simulink model "PMSM_PI_decomposition_Discrete_Time"  (R2024a)
settings: Solver=ode23tb  StartTime=0.0  StopTime=10  FixedStep=0.0002  RelTol=1e-4  EnableMultiTasking=on
InitFcn:
  | Ts = 10e-6;
  | 
  | R = 0.958;
  | Ld = 5.25e-3;
  | Lq = 12e-3;
  | Pn = 4;
  | flux = 0.1827;
values from neighbouring files (symbols this model uses):
  Flux = 0.1827    [Parameters.m]    (also in StateSpace.m = 0.192)
  Ki = (Ld*2*pi*fsw)/10    (= 2.4975661596)    [StateSpace.m]
  Kp = (Lq*2*pi*fsw)/10    (= 2.4975661596)    [StateSpace.m]
  L_d = 0.00525    [Parameters.m]
  L_q = 0.00525    [Parameters.m]
  p = 4    [Parameters.m]    (also in StateSpace.m)
  R_s = 0.9585    [Parameters.m]
undefined symbols (not defined in the file or in its folder): DiscIntNeverNeededParam, Ki_s, Kp_s
libraries: simulink x2, spsPermanentMagnetSynchronousMachineLib x1, spsUniversalBridgeLib x1, spsDCVoltageSourceLib x1, sps_lib x1
settings Model: Creator=SUN  LastModifiedBy=nicco
settings SolverCC: ZeroCrossControl=DisableAll  AlgebraicLoopSolver=TrustRegion
settings DataIOCC: LimitDataPoints=on  SaveFormat=Array  SignalLoggingSaveFormat=ModelDataLogs  ReturnWorkspaceOutputs=off
settings OptimizationCC: ExpressionDepthLimit=2147483647  InitFltsAndDblsToZero=on  LifeSpan=inf
settings DebuggingCC: UnderspecifiedInitializationDetection=Classic  MergeDetectMultiDrivingBlocksExec=none  SolverPrmCheckMsg=warning  FcnCallInpInsideContextMsg=warning  UnconnectedInputMsg=warning  UnconnectedOutputMsg=warning  UnconnectedLineMsg=warning  StateNameClashWarn=warning  SFUnexpectedBacktrackingDiag=warning  SFNoUnconditionalDefaultTransitionDiag=warning  SFExecutionAtInitializationDiag=none  ArithmeticOperatorsInVariantConditions=warning
settings HardwareCC: ProdBitPerPointer=32  ProdBitPerSizeT=32  ProdBitPerPtrDiffT=32  ProdLargestAtomicFloat=None  ProdIntDivRoundTo=Undefined  ProdEndianess=Unspecified  ProdWordSize=32  ProdHWDeviceType=32-bit Generic
settings ModelReferenceCC: EnableRefExpFcnMdlSchedulingChecks=on  PropagateSignalLabelsOutOfModel=off
settings SFSimCC: SimUseLocalCustomCode=off  CustomCodeUndefinedFunction=UseInterfaceOnly
settings RTWCC: RTWUseLocalCustomCode=off  GPUComputeCapability=3.5
settings CodeAppCC: StateflowObjectComments=on
settings GRTTargetCC: TargetLangStandard=C89/C90 (ANSI)  CombineOutputUpdateFcns=off  GRTInterface=on
settings ConfigComp: CovMetricSettings=dw  CovSaveCumulativeToWorkspaceVar=on  CovSaveSingleToWorkspaceVar=on  CovExternalEMLEnable=off  CovSFcnEnable=off
settings SimscapeCC: SimscapeNormalizeSystem=off

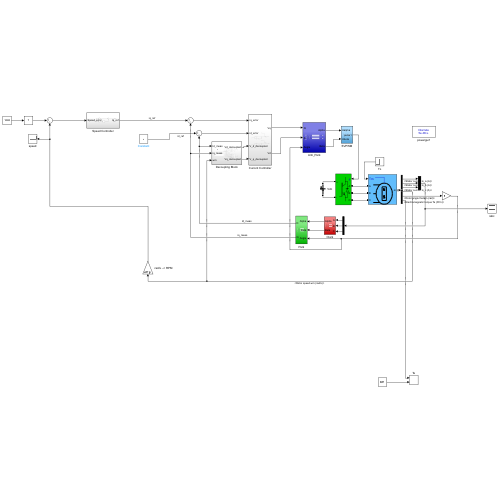
[thumbnail: Simulink's stored preview of the top-level diagram]
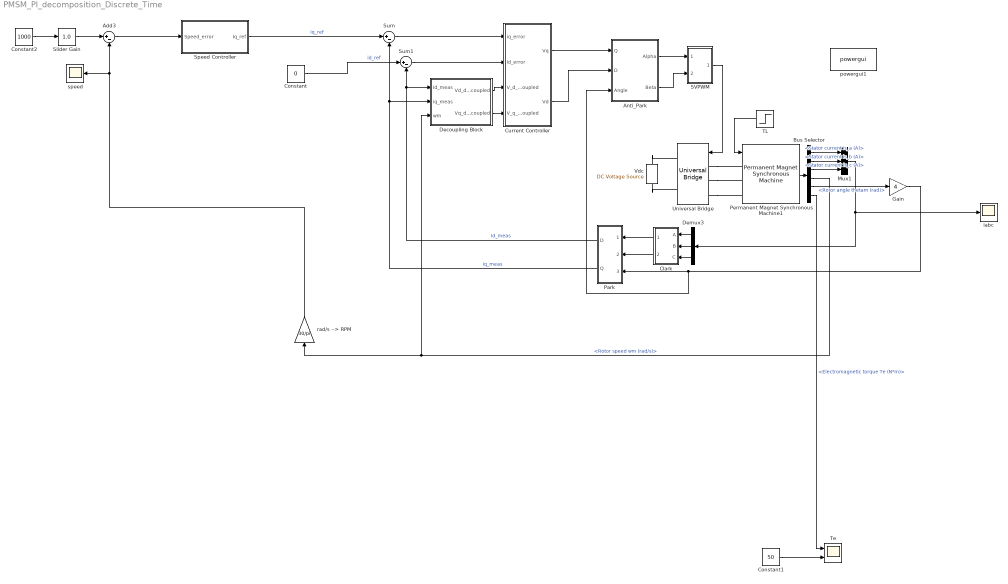
== system PMSM_PI_decomposition_Discrete_Time ==
  Add3 : Sum  Inputs=|+-
  Anti_Park : Subsystem
  Bus Selector : BusSelector  OutputSignals=Stator current is_a (A),Stator current is_b (A),Stator current is_c (A),Rotor speed wm (rad/s),Rotor angle thetam (rad),Electromagnetic torque Te (N*m)
  Clark : Subsystem
  Constant : Constant  Value=0
  Constant1 : Constant  Value=50
  Constant2 : Constant  Value=1000
  Current Controller : Subsystem
  Decoupling Block : Subsystem
  Demux3 : Demux  Outputs=3
  Gain : Gain  Gain=4
  Mux1 : Mux  Inputs=3
  Park : Subsystem
  Permanent Magnet Synchronous Machine1 : spsPermanentMagnetSynchronousMachineLib/Permanent Magnet Synchronous Machine  NbPhases=3  FluxDistribution=Sinusoidal  RotorType=Salient-pole  MechanicalLoad=Torque Tm  PresetModel=No  ShowDetailedParameters=on  MeasurementBus=off  Resistance=R_s  Inductance=8.5e-3  dqInductances=[L_d L_q]  La=L_d  MachineConstant=Flux linkage established by magnets (V.s)  Flux=Flux  VoltageCst=132.5525  TorqueCst=1.0962  Flat=120  Mechanical=[0.003 0.008 p]  PolePairs=3  InitialConditions=[0,0, 0,0]  InitialConditions5ph=[0 0 0 0 0 0]  RefAngle=Aligned with phase A axis (original Park)  IterativeDiscreteModel=Trapezoidal non iterative  TsBlock=-1  TsPowergui=0
  SVPWM : Subsystem
  Slider Gain : simulink/Math Operations/Slider Gain  gain=1.0  low=0  high=2
  Speed Controller : Subsystem
  Sum : Sum  Inputs=|+-
  Sum1 : Sum  Inputs=|+-
  TL : Step  Time=0.2  After=0  SampleTime=0
  Te : Scope  NumInputPorts=2
  Universal Bridge : spsUniversalBridgeLib/Universal Bridge  Arms=3  SnubberResistance=1e5  SnubberCapacitance=inf  Device=IGBT / Diodes  Ron=1e-3  Lon=0  ForwardVoltages="[  0  0  ]"  ForwardVoltage=0  GTOparameters=[ 10e-6 , 20e-6 ]  IGBTparameters=[ 1e-6 , 2e-6 ]  Measurements=None  Measurements_2=None  converterType=Rectifier
  Vdc : spsDCVoltageSourceLib/DC Voltage Source  Amplitude=600  Measurements=None
  iabc : Scope
  powergui1 : sps_lib/powergui  Priority=1  SimulationMode=Discrete  SampleTime=5e-6  frequency=60  Iterations=50  frequencyindice=0  Pbase=100e6  ErrMax=1e-4  UnitsV=kV  UnitsW=MW  buscounter=0  FunctionMessages=off  echomessages=off  EnableUseOfTLC=off  CurrentSourceSwitches=off  DisableSnubberDevices=off  DisableRonSwitches=off  DisableVfSwitches=off  DisplayEquations=off  AutomaticDiscreteSolvers=off  SolverType=Tustin/Backward Euler (TBE)  Interpol=off  ExternalGateDelay=off  methode=off  Ts=100  x0status=blocks  SPID=on  SwTol=0  HookPort=off  NonlinearTolerance=1e-4  nMaxIteration=100  ContinueOnMaxIteration=off  RestoreLinks=warning  ResistiveCurrentMeasurement=off  Frange=[0:2:500]  Ylog=off  Xlog=on  ShowGrid=off  save=off  variable=ZData  structure=0  ZoomFFT=off  StartTime=0.0  cycles=1  DisplayStyle=1  fundamental=60  FreqAxis=off  MaxFrequency=1000  frequencyindicesteady=1  RmsSteady=1  display=off
  rad/s --> RPM : Gain  Gain=30/pi
  speed : Scope
  wires:
  TL/1 -> Permanent Magnet Synchronous Machine1/1
  Gain/1 -> Park/3(Angle), Anti_Park/3(Angle)
  Anti_Park/1(Alpha) -> SVPWM/1(Ualpha)
  Demux3/1 -> Clark/1(A)
  Anti_Park/2(Beta) -> SVPWM/2(Ubeta)
  Demux3/2 -> Clark/2(B)
  Demux3/3 -> Clark/3(C)
  Clark/1(Alpha) -> Park/1(Alpha)
  Clark/2(Beta) -> Park/2(Beta)
  Bus Selector/3 -> Mux1/3  "<Stator current is_c (A)>"
  Bus Selector/2 -> Mux1/2  "<Stator current is_b (A)>"
  Bus Selector/1 -> Mux1/1  "<Stator current is_a (A)>"
  Mux1/1 -> iabc/1, Demux3/1
  Permanent Magnet Synchronous Machine1/1 -> Bus Selector/1
  Bus Selector/5 -> Gain/1  "<Rotor angle thetam (rad)>"
  Bus Selector/6 -> Te/1  "<Electromagnetic torque Te (N*m)>"
  SVPWM/1(pulse1) -> Universal Bridge/1
  Constant/1 -> Sum1/1  "id_ref"
  Sum/1 -> Current Controller/1(iq_error)
  Park/2(Q) -> Sum/2, Decoupling Block/2(iq_meas)  "iq_meas"
  Decoupling Block/2(Vq_decoupled) -> Current Controller/4(V_q_decoupled)
  Park/1(D) -> Sum1/2, Decoupling Block/1(Id_meas)  "Id_meas"
  Sum1/1 -> Current Controller/2(id_error)
  Decoupling Block/1(Vd_decoupled) -> Current Controller/3(V_d_decoupled)
  Bus Selector/4 -> Decoupling Block/3(wm), rad/s --> RPM/1  "<Rotor speed wm (rad/s)>"
  Current Controller/2(Vd) -> Anti_Park/2(D)
  Current Controller/1(Vq) -> Anti_Park/1(Q)
  Slider Gain/1 -> Add3/1
  rad/s --> RPM/1 -> Add3/2, speed/1
  Constant1/1 -> Te/2
  Speed Controller/1(Iq_ref) -> Sum/1  "iq_ref"
  Add3/1 -> Speed Controller/1(Speed_error)
  Constant2/1 -> Slider Gain/1
  connections:
  Universal Bridge/LConn1 -- Permanent Magnet Synchronous Machine1/LConn1
  Universal Bridge/LConn2 -- Permanent Magnet Synchronous Machine1/LConn2
  Universal Bridge/LConn3 -- Permanent Magnet Synchronous Machine1/LConn3
  Vdc/RConn1 -- Universal Bridge/RConn1
  Vdc/LConn1 -- Universal Bridge/RConn2

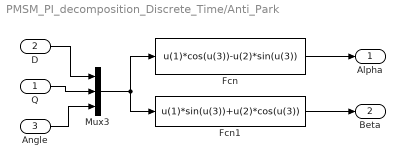
== system PMSM_PI_decomposition_Discrete_Time/Anti_Park ==
  Q : Inport
  D : Inport  Port=2
  Angle : Inport  Port=3
  Fcn : Fcn  Expr=u(1)*cos(u(3))-u(2)*sin(u(3))
  Fcn1 : Fcn  Expr=u(1)*sin(u(3))+u(2)*cos(u(3))
  Mux3 : Mux  Inputs=3
  Alpha : Outport  VectorParamsAs1DForOutWhenUnconnected=off
  Beta : Outport  Port=2  VectorParamsAs1DForOutWhenUnconnected=off
  wires:
  Angle/1 -> Mux3/3
  Fcn1/1 -> Beta/1
  Mux3/1 -> Fcn1/1, Fcn/1
  Fcn/1 -> Alpha/1
  D/1 -> Mux3/1
  Q/1 -> Mux3/2

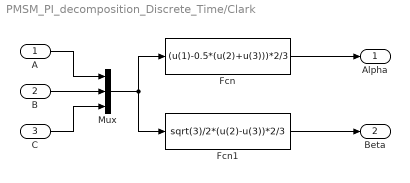
== system PMSM_PI_decomposition_Discrete_Time/Clark ==
  A : Inport
  B : Inport  Port=2
  C : Inport  Port=3
  Fcn : Fcn  Expr=(u(1)-0.5*(u(2)+u(3)))*2/3
  Fcn1 : Fcn  Expr=sqrt(3)/2*(u(2)-u(3))*2/3
  Mux : Mux  Inputs=3
  Alpha : Outport  VectorParamsAs1DForOutWhenUnconnected=off
  Beta : Outport  Port=2  VectorParamsAs1DForOutWhenUnconnected=off
  wires:
  B/1 -> Mux/2
  Mux/1 -> Fcn1/1, Fcn/1
  Fcn1/1 -> Beta/1
  Fcn/1 -> Alpha/1
  C/1 -> Mux/3
  A/1 -> Mux/1

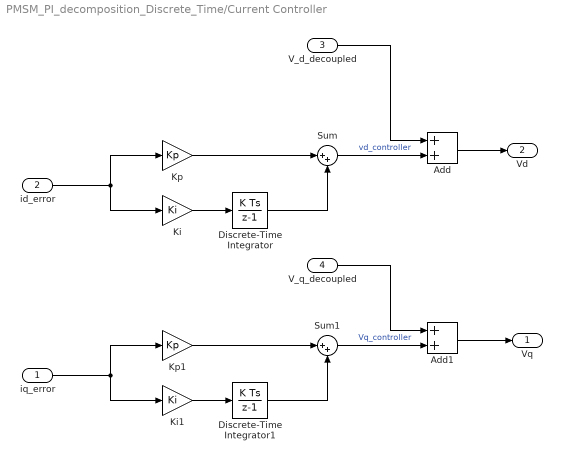
== system PMSM_PI_decomposition_Discrete_Time/Current Controller ==
  iq_error : Inport
  id_error : Inport  Port=2
  V_d_decoupled : Inport  Port=3
  V_q_decoupled : Inport  Port=4
  Add : Sum
  Add1 : Sum
  Discrete-Time Integrator : DiscreteIntegrator  SampleTime=-1  ICPrevOutput=DiscIntNeverNeededParam  ICPrevScaledInput=DiscIntNeverNeededParam
  Discrete-Time Integrator1 : DiscreteIntegrator  SampleTime=-1  ICPrevOutput=DiscIntNeverNeededParam  ICPrevScaledInput=DiscIntNeverNeededParam
  Ki : Gain  Gain=Ki
  Ki1 : Gain  Gain=Ki
  Kp : Gain  Gain=Kp
  Kp1 : Gain  Gain=Kp
  Sum : Sum  Inputs=|++
  Sum1 : Sum  Inputs=|++
  Vq : Outport
  Vd : Outport  Port=2
  wires:
  Add/1 -> Vd/1
  id_error/1 -> Ki/1, Kp/1
  V_q_decoupled/1 -> Add1/1
  Ki1/1 -> Discrete-Time Integrator1/1
  V_d_decoupled/1 -> Add/1
  iq_error/1 -> Ki1/1, Kp1/1
  Kp1/1 -> Sum1/1
  Sum/1 -> Add/2  "vd_controller"
  Sum1/1 -> Add1/2  "Vq_controller"
  Discrete-Time Integrator1/1 -> Sum1/2
  Discrete-Time Integrator/1 -> Sum/2
  Ki/1 -> Discrete-Time Integrator/1
  Kp/1 -> Sum/1
  Add1/1 -> Vq/1

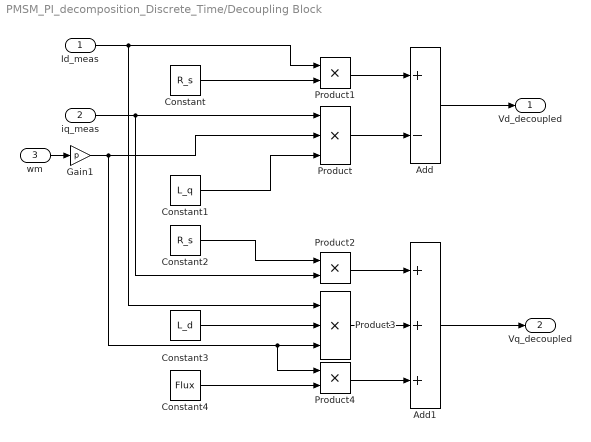
== system PMSM_PI_decomposition_Discrete_Time/Decoupling Block ==
  Id_meas : Inport
  iq_meas : Inport  Port=2
  wm : Inport  Port=3
  Add : Sum  Inputs=+-
  Add1 : Sum  Inputs=+++
  Constant : Constant  Value=R_s
  Constant1 : Constant  Value=L_q
  Constant2 : Constant  Value=R_s
  Constant3 : Constant  Value=L_d
  Constant4 : Constant  Value=Flux
  Gain1 : Gain  Gain=p
  Product : Product  Inputs=3
  Product1 : Product
  Product2 : Product
  Product3 : Product  Inputs=3
  Product4 : Product
  Vd_decoupled : Outport
  Vq_decoupled : Outport  Port=2
  wires:
  Add/1 -> Vd_decoupled/1
  Product1/1 -> Add/1
  Constant/1 -> Product1/2
  Id_meas/1 -> Product1/1, Product3/1
  Product/1 -> Add/2
  Gain1/1 -> Product4/1, Product3/3, Product/2
  Constant1/1 -> Product/3
  Add1/1 -> Vq_decoupled/1
  Product2/1 -> Add1/1
  Constant2/1 -> Product2/1
  iq_meas/1 -> Product/1, Product2/2
  Product3/1 -> Add1/2
  Constant3/1 -> Product3/2
  Product4/1 -> Add1/3
  Constant4/1 -> Product4/2
  wm/1 -> Gain1/1

== system PMSM_PI_decomposition_Discrete_Time/Park ==
  Alpha : Inport
  Beta : Inport  Port=2
  Angle : Inport  Port=3
  Fcn : Fcn  Expr=u(1)*cos(u(3))+u(2)*sin(u(3))
  Fcn1 : Fcn  Expr=u(2)*cos(u(3))-u(1)*sin(u(3))
  Mux2 : Mux  Inputs=3
  D : Outport  VectorParamsAs1DForOutWhenUnconnected=off
  Q : Outport  Port=2  VectorParamsAs1DForOutWhenUnconnected=off
  wires:
  Beta/1 -> Mux2/2
  Mux2/1 -> Fcn1/1, Fcn/1
  Angle/1 -> Mux2/3
  Alpha/1 -> Mux2/1
  Fcn1/1 -> Q/1
  Fcn/1 -> D/1

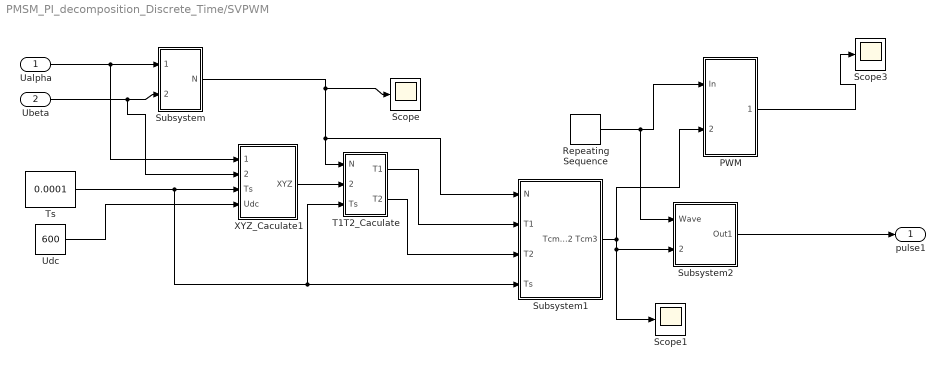
== system PMSM_PI_decomposition_Discrete_Time/SVPWM ==
  Ualpha : Inport
  Ubeta : Inport  Port=2
  PWM : Subsystem
  Repeating Sequence : simulink/Sources/Repeating Sequence  rep_seq_t=[0 0.00005 0.0001]  rep_seq_y=[0 0.00005 0]
  Scope : Scope
  Scope1 : Scope
  Scope3 : Scope
  Subsystem : Subsystem
  Subsystem1 : Subsystem
  Subsystem2 : Subsystem
  T1T2_Caculate : Subsystem
  Ts : Constant  Value=0.0001
  Udc : Constant  Value=600
  XYZ_Caculate1 : Subsystem
  pulse1 : Outport  VectorParamsAs1DForOutWhenUnconnected=off
  wires:
  T1T2_Caculate/1(T1) -> Subsystem1/2(T1)
  Ts/1 -> XYZ_Caculate1/3(Ts), T1T2_Caculate/3(Ts), Subsystem1/4(Ts)
  Udc/1 -> XYZ_Caculate1/4(Udc)
  Subsystem/1(N) -> Scope/1, T1T2_Caculate/1(N), Subsystem1/1(N)
  T1T2_Caculate/2(T2) -> Subsystem1/3(T2)
  XYZ_Caculate1/1("XYZ ") -> T1T2_Caculate/2(XYZ)
  Ualpha/1 -> XYZ_Caculate1/1(Ualpha), Subsystem/1(Ualpha)
  Ubeta/1 -> XYZ_Caculate1/2(Ubeta), Subsystem/2(Ubeta)
  Subsystem1/1(Tcm1 Tcm2 Tcm3) -> Scope1/1, Subsystem2/2(Tcm123), PWM/2(Tcm123)
  Repeating Sequence/1 -> Subsystem2/1(Wave), PWM/1(In)
  PWM/1(PWM) -> Scope3/1
  Subsystem2/1(Out1) -> pulse1/1

== system PMSM_PI_decomposition_Discrete_Time/Speed Controller ==
  Speed_error : Inport
  Discrete-Time Integrator : DiscreteIntegrator  SampleTime=-1  ICPrevOutput=DiscIntNeverNeededParam  ICPrevScaledInput=DiscIntNeverNeededParam
  Ki : Gain  Gain=Ki_s
  Kp : Gain  Gain=Kp_s
  Sum2 : Sum  Inputs=|++
  Iq_ref : Outport
  wires:
  Discrete-Time Integrator/1 -> Sum2/2
  Sum2/1 -> Iq_ref/1  "vd_controller"
  Kp/1 -> Sum2/1
  Speed_error/1 -> Ki/1, Kp/1
  Ki/1 -> Discrete-Time Integrator/1

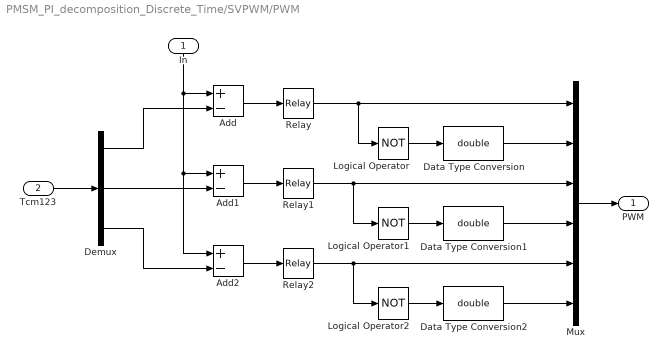
== system PMSM_PI_decomposition_Discrete_Time/SVPWM/PWM ==
  In : Inport
  Tcm123 : Inport  Port=2
  Add : Sum  Inputs=+-
  Add1 : Sum  Inputs=+-
  Add2 : Sum  Inputs=+-
  Data Type Conversion : DataTypeConversion  OutDataTypeStr=double  SaturateOnIntegerOverflow=off  RndMeth=Floor
  Data Type Conversion1 : DataTypeConversion  OutDataTypeStr=double  SaturateOnIntegerOverflow=off  RndMeth=Floor
  Data Type Conversion2 : DataTypeConversion  OutDataTypeStr=double  SaturateOnIntegerOverflow=off  RndMeth=Floor
  Demux : Demux  Outputs=3
  Logical Operator : Logic  Operator=NOT  AllPortsSameDT=off  OutDataTypeStr=boolean
  Logical Operator1 : Logic  Operator=NOT  AllPortsSameDT=off  OutDataTypeStr=boolean
  Logical Operator2 : Logic  Operator=NOT  AllPortsSameDT=off  OutDataTypeStr=boolean
  Mux : Mux  Inputs=6
  Relay : Relay  OffSwitchValue=-eps
  Relay1 : Relay  OffSwitchValue=-eps
  Relay2 : Relay  OffSwitchValue=-eps
  PWM : Outport  VectorParamsAs1DForOutWhenUnconnected=off
  wires:
  Demux/3 -> Add2/2
  Demux/2 -> Add1/2
  Demux/1 -> Add/2
  Relay2/1 -> Mux/5, Logical Operator2/1
  Relay1/1 -> Mux/3, Logical Operator1/1
  Relay/1 -> Logical Operator/1, Mux/1
  Mux/1 -> PWM/1
  Data Type Conversion/1 -> Mux/2
  Data Type Conversion1/1 -> Mux/4
  Data Type Conversion2/1 -> Mux/6
  Logical Operator2/1 -> Data Type Conversion2/1
  Logical Operator1/1 -> Data Type Conversion1/1
  Logical Operator/1 -> Data Type Conversion/1
  Add1/1 -> Relay1/1
  Add2/1 -> Relay2/1
  Add/1 -> Relay/1
  In/1 -> Add/1, Add2/1, Add1/1
  Tcm123/1 -> Demux/1

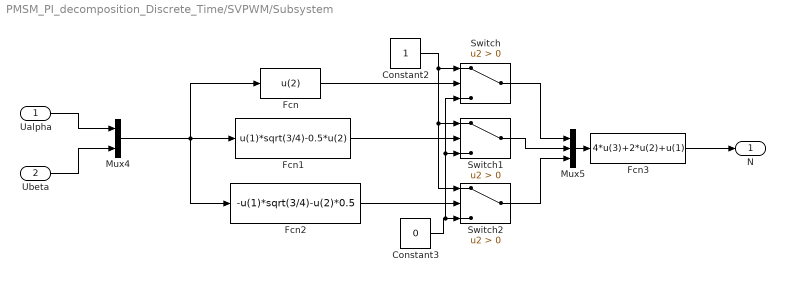
== system PMSM_PI_decomposition_Discrete_Time/SVPWM/Subsystem ==
  Ualpha : Inport
  Ubeta : Inport  Port=2
  Constant2 : Constant
  Constant3 : Constant  Value=0
  Fcn : Fcn  Expr=u(2)
  Fcn1 : Fcn  Expr=u(1)*sqrt(3/4)-0.5*u(2)
  Fcn2 : Fcn  Expr=-u(1)*sqrt(3/4)-u(2)*0.5
  Fcn3 : Fcn  Expr=4*u(3)+2*u(2)+u(1)
  Mux4 : Mux  Inputs=2
  Mux5 : Mux  Inputs=3
  Switch : Switch  Criteria=u2 > Threshold  SaturateOnIntegerOverflow=off  InputSameDT=off
  Switch1 : Switch  Criteria=u2 > Threshold  SaturateOnIntegerOverflow=off  InputSameDT=off
  Switch2 : Switch  Criteria=u2 > Threshold  SaturateOnIntegerOverflow=off  InputSameDT=off
  N : Outport  VectorParamsAs1DForOutWhenUnconnected=off
  wires:
  Switch/1 -> Mux5/1
  Ualpha/1 -> Mux4/1
  Constant2/1 -> Switch2/1, Switch1/1, Switch/1
  Mux4/1 -> Fcn/1, Fcn2/1, Fcn1/1
  Fcn2/1 -> Switch2/2
  Ubeta/1 -> Mux4/2
  Fcn3/1 -> N/1
  Constant3/1 -> Switch/3, Switch1/3, Switch2/3
  Fcn/1 -> Switch/2
  Switch2/1 -> Mux5/3
  Fcn1/1 -> Switch1/2
  Switch1/1 -> Mux5/2
  Mux5/1 -> Fcn3/1

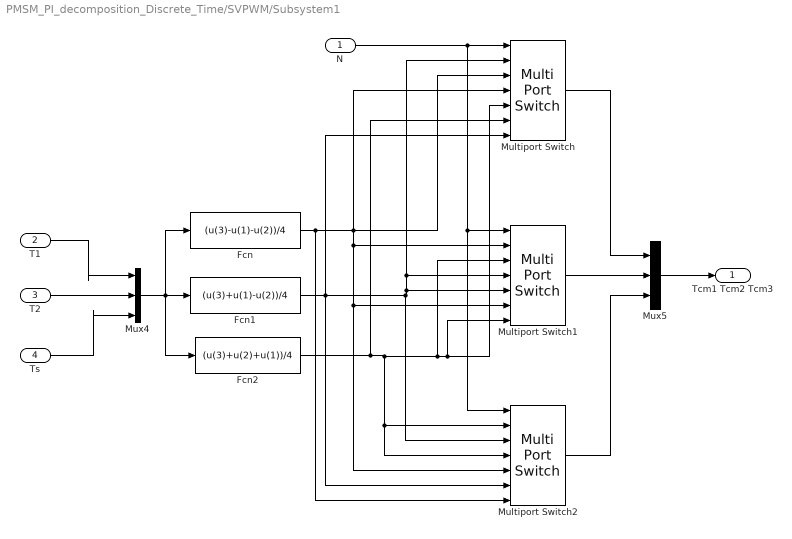
== system PMSM_PI_decomposition_Discrete_Time/SVPWM/Subsystem1 ==
  N : Inport
  T1 : Inport  Port=2
  T2 : Inport  Port=3
  Ts : Inport  Port=4
  Fcn : Fcn  Expr=(u(3)-u(1)-u(2))/4
  Fcn1 : Fcn  Expr=(u(3)+u(1)-u(2))/4
  Fcn2 : Fcn  Expr=(u(3)+u(2)+u(1))/4
  Multiport Switch : MultiPortSwitch  Inputs=6  SaturateOnIntegerOverflow=off  InputSameDT=off
  Multiport Switch1 : MultiPortSwitch  Inputs=6  SaturateOnIntegerOverflow=off  InputSameDT=off
  Multiport Switch2 : MultiPortSwitch  Inputs=6  SaturateOnIntegerOverflow=off  InputSameDT=off
  Mux4 : Mux  Inputs=3
  Mux5 : Mux  Inputs=3
  Tcm1 Tcm2 Tcm3 : Outport  VectorParamsAs1DForOutWhenUnconnected=off
  wires:
  T2/1 -> Mux4/2
  N/1 -> Multiport Switch2/1, Multiport Switch1/1, Multiport Switch/1
  Mux5/1 -> Tcm1 Tcm2 Tcm3/1
  T1/1 -> Mux4/1
  Fcn1/1 -> Multiport Switch/7, Multiport Switch2/6, Multiport Switch2/3, Multiport Switch1/5, Multiport Switch1/4, Multiport Switch/2
  Mux4/1 -> Fcn2/1, Fcn1/1, Fcn/1
  Multiport Switch2/1 -> Mux5/3
  Fcn/1 -> Multiport Switch2/7, Multiport Switch1/6, Multiport Switch2/5, Multiport Switch1/2, Multiport Switch/3, Multiport Switch/4
  Multiport Switch1/1 -> Mux5/2
  Fcn2/1 -> Multiport Switch/6, Multiport Switch1/7, Multiport Switch/5, Multiport Switch1/3, Multiport Switch2/4, Multiport Switch2/2
  Ts/1 -> Mux4/3
  Multiport Switch/1 -> Mux5/1

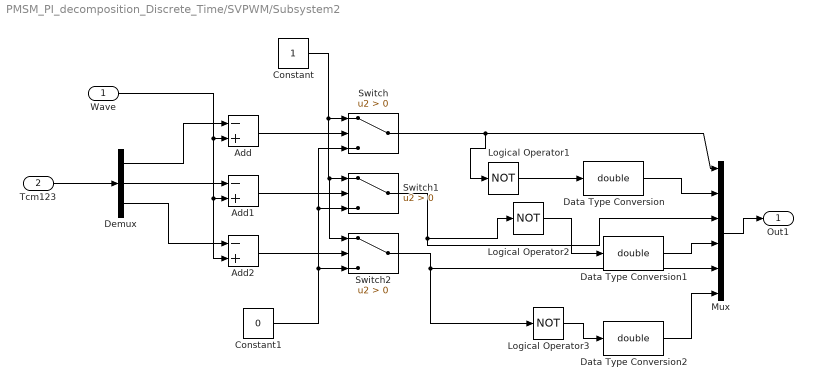
== system PMSM_PI_decomposition_Discrete_Time/SVPWM/Subsystem2 ==
  Wave : Inport
  Tcm123 : Inport  Port=2
  Add : Sum  Inputs=-+
  Add1 : Sum  Inputs=-+
  Add2 : Sum  Inputs=-+
  Constant : Constant
  Constant1 : Constant  Value=0
  Data Type Conversion : DataTypeConversion  OutDataTypeStr=double  SaturateOnIntegerOverflow=off  RndMeth=Floor
  Data Type Conversion1 : DataTypeConversion  OutDataTypeStr=double  SaturateOnIntegerOverflow=off  RndMeth=Floor
  Data Type Conversion2 : DataTypeConversion  OutDataTypeStr=double  SaturateOnIntegerOverflow=off  RndMeth=Floor
  Demux : Demux  Outputs=3
  Logical Operator1 : Logic  Operator=NOT  AllPortsSameDT=off  OutDataTypeStr=boolean
  Logical Operator2 : Logic  Operator=NOT  AllPortsSameDT=off  OutDataTypeStr=boolean
  Logical Operator3 : Logic  Operator=NOT  AllPortsSameDT=off  OutDataTypeStr=boolean
  Mux : Mux  Inputs=6
  Switch : Switch  Criteria=u2 > Threshold  SaturateOnIntegerOverflow=off  InputSameDT=off
  Switch1 : Switch  Criteria=u2 > Threshold  SaturateOnIntegerOverflow=off  InputSameDT=off
  Switch2 : Switch  Criteria=u2 > Threshold  SaturateOnIntegerOverflow=off  InputSameDT=off
  Out1 : Outport  VectorParamsAs1DForOutWhenUnconnected=off
  wires:
  Add2/1 -> Switch2/2
  Add1/1 -> Switch1/2
  Constant/1 -> Switch2/1, Switch1/1, Switch/1
  Switch/1 -> Logical Operator1/1, Mux/1
  Wave/1 -> Add2/2, Add1/2, Add/2
  Demux/3 -> Add2/1
  Constant1/1 -> Switch2/3, Switch1/3, Switch/3
  Add/1 -> Switch/2
  Switch1/1 -> Mux/3, Logical Operator2/1
  Switch2/1 -> Mux/5, Logical Operator3/1
  Demux/1 -> Add/1
  Tcm123/1 -> Demux/1
  Demux/2 -> Add1/1
  Mux/1 -> Out1/1
  Logical Operator1/1 -> Data Type Conversion/1
  Data Type Conversion/1 -> Mux/2
  Data Type Conversion1/1 -> Mux/4
  Logical Operator2/1 -> Data Type Conversion1/1
  Data Type Conversion2/1 -> Mux/6
  Logical Operator3/1 -> Data Type Conversion2/1

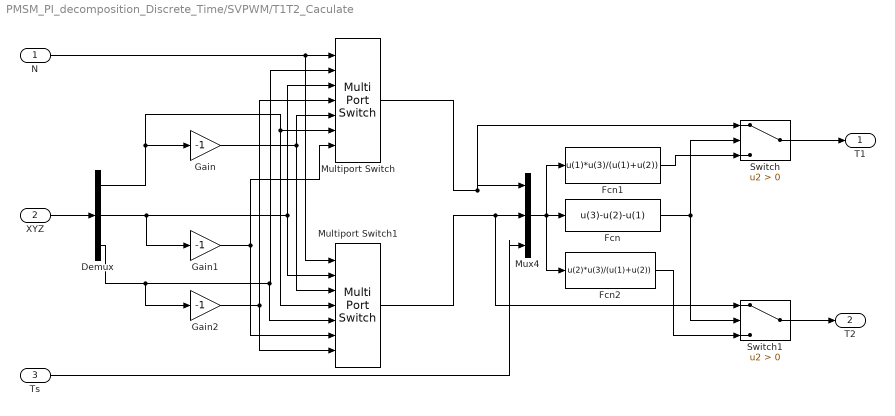
== system PMSM_PI_decomposition_Discrete_Time/SVPWM/T1T2_Caculate ==
  N : Inport
  XYZ : Inport  Port=2
  Ts : Inport  Port=3
  Demux : Demux  Outputs=3
  Fcn : Fcn  Expr=u(3)-u(2)-u(1)
  Fcn1 : Fcn  Expr=u(1)*u(3)/(u(1)+u(2))
  Fcn2 : Fcn  Expr=u(2)*u(3)/(u(1)+u(2))
  Gain : Gain  Gain=-1
  Gain1 : Gain  Gain=-1
  Gain2 : Gain  Gain=-1
  Multiport Switch : MultiPortSwitch  Inputs=6  SaturateOnIntegerOverflow=off  InputSameDT=off
  Multiport Switch1 : MultiPortSwitch  Inputs=6  SaturateOnIntegerOverflow=off  InputSameDT=off
  Mux4 : Mux  Inputs=3
  Switch : Switch  Criteria=u2 > Threshold  SaturateOnIntegerOverflow=off  InputSameDT=off
  Switch1 : Switch  Criteria=u2 > Threshold  SaturateOnIntegerOverflow=off  InputSameDT=off
  T1 : Outport  VectorParamsAs1DForOutWhenUnconnected=off
  T2 : Outport  Port=2  VectorParamsAs1DForOutWhenUnconnected=off
  wires:
  Gain1/1 -> Multiport Switch/7, Multiport Switch1/6
  Fcn2/1 -> Switch1/3
  Demux/2 -> Gain1/1, Multiport Switch/3, Multiport Switch1/2
  Demux/3 -> Multiport Switch1/5, Multiport Switch/2, Gain2/1
  N/1 -> Multiport Switch1/1, Multiport Switch/1
  Demux/1 -> Gain/1, Multiport Switch/6, Multiport Switch1/4
  Mux4/1 -> Fcn2/1, Fcn1/1, Fcn/1
  XYZ/1 -> Demux/1
  Gain/1 -> Multiport Switch1/3, Multiport Switch/5
  Fcn/1 -> Switch1/2, Switch/2
  Multiport Switch1/1 -> Switch1/1, Mux4/2
  Fcn1/1 -> Switch/3
  Multiport Switch/1 -> Switch/1, Mux4/1
  Gain2/1 -> Multiport Switch1/7, Multiport Switch/4
  Switch1/1 -> T2/1
  Ts/1 -> Mux4/3
  Switch/1 -> T1/1

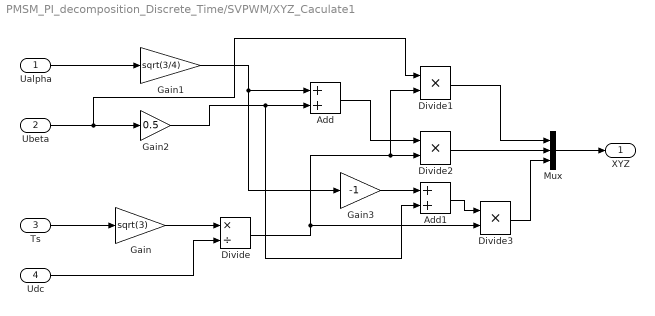
== system PMSM_PI_decomposition_Discrete_Time/SVPWM/XYZ_Caculate1 ==
  Ualpha : Inport
  Ubeta : Inport  Port=2
  Ts : Inport  Port=3
  Udc : Inport  Port=4
  Add : Sum
  Add1 : Sum
  Divide : Product  Inputs=*/
  Divide1 : Product  Inputs=**
  Divide2 : Product  Inputs=**
  Divide3 : Product  Inputs=**
  Gain : Gain  Gain=sqrt(3)
  Gain1 : Gain  Gain=sqrt(3/4)
  Gain2 : Gain  Gain=0.5
  Gain3 : Gain  Gain=-1
  Mux : Mux  Inputs=3
  "XYZ " : Outport  VectorParamsAs1DForOutWhenUnconnected=off
  wires:
  Mux/1 -> "XYZ "/1
  Divide2/1 -> Mux/2
  Divide1/1 -> Mux/1
  Gain/1 -> Divide/1
  Udc/1 -> Divide/2
  Ualpha/1 -> Gain1/1
  Add/1 -> Divide2/1
  Divide/1 -> Divide3/2, Divide2/2, Divide1/2
  Gain3/1 -> Add1/1
  Ubeta/1 -> Divide1/1, Gain2/1
  Gain1/1 -> Add/1, Gain3/1
  Gain2/1 -> Add/2, Add1/2
  Ts/1 -> Gain/1
  Add1/1 -> Divide3/1
  Divide3/1 -> Mux/3
